simulink library "sm_motor_grader_lib"  (R2026a)
settings: Solver=VariableStepAuto
undefined symbols (not defined in the file): activeTestCmds, Art, Center, Circle, Driver, HMPST, LiftL, LiftR, LnL, LnR, Loads, Maneuver, motGradParams, Pin, RFL, RFR, RRL, RRR, SceneData, Side, Sphere, StrL, StrR, Tilt, X, Y, Z
libraries: sm_lib x219, nesl_utility x134, fl_lib x53, $bdroot x24, cvt_powertrain_lib x6, simulink_extras x5, grid_element x4, simulink x3, cvt_powertrain_lib_vnts x3, Driver_Long_Lat_Stanley x1, Maneuver_Get_Pose x1, SignalEditorBlockLib x1
(part 7 of 13)

== system sm_motor_grader_lib/Powertrain/Torque4 ==
  BusElementIn : Inport  PortName=Cmd  Element=vVeh
  BusElementIn1 : Inport  Port=2  PortName=m  Element=FrameR.Body.Ref.vx
  Gain : Gain  Gain=motGradParams.drivetrain.propGain
  Gain1 : Gain  Gain=motGradParams.drivetrain.integral
  Gain2 : Gain  Gain=4
  Integrator : Integrator
  Mechanical Rotational Reference : fl_lib/Mechanical/Rotational Elements/Mechanical Rotational Reference
  Simscape Bus : SimscapeBus  HierarchyStrings=RFL;RFR;RRL;RRR
  Simulink-PS Converter{,1..3} (4 alike) : nesl_utility/Simulink-PS Converter  PhysicalDomain=network_engine_domain  SubClassName=ps_input  LeftPortType=input  RightPortType=output  PseudoPeriodic=off  Frequencies=[]  NoiseDistribution=none  NoiseParameters=[]  Unit=1  AffineConversion=off  FilteringAndDerivatives=provide  SimscapeFilterOrder=1  InputFilterTimeConstant=0.001  UdotUserProvided=0
  Subtract : Sum  Inputs=+-
  Sum : Sum  Inputs=|++
  Torque Source FL : fl_lib/Mechanical/Mechanical Sources/Ideal Torque Source
  Torque Source FR : fl_lib/Mechanical/Mechanical Sources/Ideal Torque Source
  Torque Source RL : fl_lib/Mechanical/Mechanical Sources/Ideal Torque Source
  Torque Source RR : fl_lib/Mechanical/Mechanical Sources/Ideal Torque Source
  Dtr : PMIOPort  Side=Right
  Out Bus Element : Outport  PortName=meas  Element=trqDrv
  wires:
  BusElementIn/1 -> Subtract/1
  Subtract/1 -> Gain1/1, Gain/1
  Gain1/1 -> Integrator/1
  Gain/1 -> Sum/1
  Integrator/1 -> Sum/2
  Sum/1 -> Simulink-PS Converter1/1, Simulink-PS Converter/1, Gain2/1, Simulink-PS Converter2/1, Simulink-PS Converter3/1
  BusElementIn1/1 -> Subtract/2
  Gain2/1 -> Out Bus Element/1
  connections:
  Torque Source FL/RConn2 -- Torque Source FR/RConn2 -- Mechanical Rotational Reference/LConn1 -- Torque Source RR/RConn2 -- Torque Source RL/RConn2
  Simulink-PS Converter2/RConn1 -- Torque Source RL/RConn1
  Simulink-PS Converter/RConn1 -- Torque Source FL/RConn1
  Torque Source RL/LConn1 -- Simscape Bus/LConn3
  Simulink-PS Converter3/RConn1 -- Torque Source RR/RConn1
  Torque Source RR/LConn1 -- Simscape Bus/LConn4
  Simulink-PS Converter1/RConn1 -- Torque Source FR/RConn1
  Torque Source FL/LConn1 -- Simscape Bus/LConn1
  Torque Source FR/LConn1 -- Simscape Bus/LConn2
  Dtr/RConn1 -- Simscape Bus/RConn1

== system sm_motor_grader_lib/Surface/Bank ==
  Bank : grid_element/Grid  VariantControl=Grid  grid_x=SceneData.bank.grid.len  grid_y=SceneData.bank.grid.wid  grid_z=SceneData.bank.grid.dep  grid_line_width=SceneData.bank.grid.line_wid  grid_num_sq_x=SceneData.bank.grid.nsq_x  grid_num_sq_y=SceneData.bank.grid.nsq_y  grid_clr=SceneData.bank.grid.line_clr  plane_clr=SceneData.bank.grid.surf_clr  grid_opc=SceneData.bank.grid.line_opc  plane_opc=SceneData.bank.grid.surf_opc
  Grid : grid_element/Grid  VariantControl=Grid  grid_x=SceneData.grid.len  grid_y=SceneData.grid.wid  grid_z=SceneData.grid.dep  grid_line_width=SceneData.grid.line_wid  grid_num_sq_x=SceneData.grid.nsq_x  grid_num_sq_y=SceneData.grid.nsq_y  grid_clr=SceneData.grid.line_clr  plane_clr=SceneData.bank.grid.surf_clr  grid_opc=SceneData.grid.line_opc  plane_opc=SceneData.grid.surf_opc
  Grid Surface : sm_lib/Curves and Surfaces/Grid Surface  XGridVector=SceneData.bank.x_vec  XGridVectorUnits=m  YGridVector=SceneData.bank.y_vec  YGridVectorUnits=m  ZHeights=SceneData.bank.z_mat  ZHeightsUnits=m  GraphicType=None  GraphicVisPropType=SimpleVisualProperties  GraphicDiffuseColor=SceneData.bank.clr  GraphicOpacity=1  GraphicSpecularColor=[0.5 0.5 0.5 1.0]  GraphicAmbientColor=[0.15 0.15 0.15 1.0]  GraphicEmissiveColor=[0.0 0.0 0.0 1.0]  GraphicShininess=75
  Spline : sm_lib/Curves and Surfaces/Spline  DataPoints=[Maneuver.Trajectory.x.Value;Maneuver.Trajectory.y.Value;Maneuver.Trajectory.zbank.Value]'  DataPointsUnits=m  EndConditionType=Natural  GraphicType=FromGeometry  MarkerShape=Sphere  MarkerSize=10  GraphicVisPropType=SimpleVisualProperties  GraphicDiffuseColor=[0 0 0]  GraphicOpacity=1  GraphicSpecularColor=[0.5 0.5 0.5 1.0]  GraphicAmbientColor=[0.15 0.15 0.15 1.0]  GraphicEmissiveColor=[0.0 0.0 0.0 1.0]  GraphicShininess=75
  Transform Offset Bank : sm_lib/Frames and Transforms/Rigid Transform  RotationMethod=StandardAxis  FollAlignAxisA=+X  BaseAlignAxisA=+Y  FollAlignAxisB=+Y  BaseAlignAxisB=+Z  RotationStandardAxis=+X  RotationAngle=SceneData.bank.qBank  RotationAngleUnits=deg  RotationArbitraryAxis=[0 0 1]  RotationSequenceAxes=FollowerAxes  RotationSequence=XYX  RotationSequenceAngles=[0 0 0]  RotationSequenceAnglesUnits=deg  RotationMatrix=[1 0 0;0 1 0;0 0 1]  Quaternion=[1 0 0 0]  TranslationMethod=Cartesian  TranslationCartesianOffset=SceneData.bank.offset  TranslationCartesianOffsetUnits=m  TranslationStandardAxis=+X  TranslationStandardOffset=SceneData.grid.len/2-10  TranslationStandardOffsetUnits=m  TranslationROffset=0  TranslationROffsetUnits=m  TranslationThetaOffset=0  TranslationThetaOffsetUnits=deg  TranslationZOffset=0  TranslationZOffsetUnits=m
  Transform Offset Grid : sm_lib/Frames and Transforms/Rigid Transform  RotationMethod=None  FollAlignAxisA=+X  BaseAlignAxisA=+Y  FollAlignAxisB=+Y  BaseAlignAxisB=+Z  RotationStandardAxis=+Z  RotationAngle=0  RotationAngleUnits=deg  RotationArbitraryAxis=[0 0 1]  RotationSequenceAxes=FollowerAxes  RotationSequence=XYX  RotationSequenceAngles=[0 0 0]  RotationSequenceAnglesUnits=deg  RotationMatrix=[1 0 0;0 1 0;0 0 1]  Quaternion=[1 0 0 0]  TranslationMethod=StandardAxis  TranslationCartesianOffset=[0 0 0]  TranslationCartesianOffsetUnits=m  TranslationStandardAxis=+X  TranslationStandardOffset=SceneData.grid.len/2-10  TranslationStandardOffsetUnits=m  TranslationROffset=0  TranslationROffsetUnits=m  TranslationThetaOffset=0  TranslationThetaOffsetUnits=deg  TranslationZOffset=0  TranslationZOffsetUnits=m
  G : PMIOPort  Side=Right
  W : PMIOPort  Port=2  Side=Left
  connections:
  G/RConn1 -- Grid Surface/RConn1
  Transform Offset Grid/LConn1 -- Spline/LConn1 -- W/RConn1
  Grid/RConn1 -- Transform Offset Bank/LConn1 -- Grid Surface/LConn1 -- Transform Offset Grid/RConn1
  Bank/RConn1 -- Transform Offset Bank/RConn1

== system sm_motor_grader_lib/Surface/Grid ==
  Grid : grid_element/Grid  VariantControl=Grid  grid_x=SceneData.grid.len  grid_y=SceneData.grid.wid  grid_z=SceneData.grid.dep  grid_line_width=SceneData.grid.line_wid  grid_num_sq_x=SceneData.grid.nsq_x  grid_num_sq_y=SceneData.grid.nsq_y  grid_clr=SceneData.grid.line_clr  plane_clr=SceneData.grid.surf_clr  grid_opc=SceneData.grid.line_opc  plane_opc=SceneData.grid.surf_opc
  Infinite Plane : sm_lib/Curves and Surfaces/Infinite Plane  GraphicType=None  GraphicPlaneWidth=10  GraphicPlaneWidthUnits=m  GraphicPlaneHeight=10  GraphicPlaneHeightUnits=m  GraphicVisPropType=SimpleVisualProperties  GraphicDiffuseColor=[0.8 0.8 0.8]  GraphicOpacity=0.7  GraphicSpecularColor=[0.5 0.5 0.5 1.0]  GraphicAmbientColor=[0.15 0.15 0.15 1.0]  GraphicEmissiveColor=[0.0 0.0 0.0 1.0]  GraphicShininess=75
  Spline : sm_lib/Curves and Surfaces/Spline  DataPoints=[Maneuver.Trajectory.x.Value;Maneuver.Trajectory.y.Value;Maneuver.Trajectory.zgrid.Value]'  DataPointsUnits=m  EndConditionType=Natural  GraphicType=FromGeometry  MarkerShape=Sphere  MarkerSize=10  GraphicVisPropType=SimpleVisualProperties  GraphicDiffuseColor=[0 0 0]  GraphicOpacity=1  GraphicSpecularColor=[0.5 0.5 0.5 1.0]  GraphicAmbientColor=[0.15 0.15 0.15 1.0]  GraphicEmissiveColor=[0.0 0.0 0.0 1.0]  GraphicShininess=75
  Transform Offset Grid : sm_lib/Frames and Transforms/Rigid Transform  RotationMethod=None  FollAlignAxisA=+X  BaseAlignAxisA=+Y  FollAlignAxisB=+Y  BaseAlignAxisB=+Z  RotationStandardAxis=+Z  RotationAngle=0  RotationAngleUnits=deg  RotationArbitraryAxis=[0 0 1]  RotationSequenceAxes=FollowerAxes  RotationSequence=XYX  RotationSequenceAngles=[0 0 0]  RotationSequenceAnglesUnits=deg  RotationMatrix=[1 0 0;0 1 0;0 0 1]  Quaternion=[1 0 0 0]  TranslationMethod=StandardAxis  TranslationCartesianOffset=[0 0 0]  TranslationCartesianOffsetUnits=m  TranslationStandardAxis=+X  TranslationStandardOffset=SceneData.grid.len/2-10  TranslationStandardOffsetUnits=m  TranslationROffset=0  TranslationROffsetUnits=m  TranslationThetaOffset=0  TranslationThetaOffsetUnits=deg  TranslationZOffset=0  TranslationZOffsetUnits=m
  G : PMIOPort  Side=Right
  W : PMIOPort  Port=2  Side=Left
  connections:
  Grid/RConn1 -- Transform Offset Grid/RConn1
  W/RConn1 -- Spline/LConn1 -- Transform Offset Grid/LConn1 -- Infinite Plane/LConn1
  G/RConn1 -- Infinite Plane/RConn1

== system sm_motor_grader_lib/Surface/Parked ==
  Grid : grid_element/Grid  VariantControl=Grid  grid_x=SceneData.park.len  grid_y=SceneData.park.wid  grid_z=SceneData.park.dep  grid_line_width=SceneData.park.line_wid  grid_num_sq_x=SceneData.park.nsq_x  grid_num_sq_y=SceneData.park.nsq_y  grid_clr=SceneData.park.line_clr  plane_clr=SceneData.park.surf_clr  grid_opc=SceneData.park.line_opc  plane_opc=SceneData.park.surf_opc
  Infinite Plane : sm_lib/Curves and Surfaces/Infinite Plane  GraphicType=None  GraphicPlaneWidth=10  GraphicPlaneWidthUnits=m  GraphicPlaneHeight=10  GraphicPlaneHeightUnits=m  GraphicVisPropType=SimpleVisualProperties  GraphicDiffuseColor=[0.8 0.8 0.8]  GraphicOpacity=0.7  GraphicSpecularColor=[0.5 0.5 0.5 1.0]  GraphicAmbientColor=[0.15 0.15 0.15 1.0]  GraphicEmissiveColor=[0.0 0.0 0.0 1.0]  GraphicShininess=75
  Transform Offset Grid : sm_lib/Frames and Transforms/Rigid Transform  RotationMethod=None  FollAlignAxisA=+X  BaseAlignAxisA=+Y  FollAlignAxisB=+Y  BaseAlignAxisB=+Z  RotationStandardAxis=+Z  RotationAngle=0  RotationAngleUnits=deg  RotationArbitraryAxis=[0 0 1]  RotationSequenceAxes=FollowerAxes  RotationSequence=XYX  RotationSequenceAngles=[0 0 0]  RotationSequenceAnglesUnits=deg  RotationMatrix=[1 0 0;0 1 0;0 0 1]  Quaternion=[1 0 0 0]  TranslationMethod=StandardAxis  TranslationCartesianOffset=[0 0 0]  TranslationCartesianOffsetUnits=m  TranslationStandardAxis=+X  TranslationStandardOffset=SceneData.park.len/2-10  TranslationStandardOffsetUnits=m  TranslationROffset=0  TranslationROffsetUnits=m  TranslationThetaOffset=0  TranslationThetaOffsetUnits=deg  TranslationZOffset=0  TranslationZOffsetUnits=m
  G : PMIOPort  Side=Right
  W : PMIOPort  Port=2  Side=Left
  connections:
  G/RConn1 -- Infinite Plane/RConn1
  Infinite Plane/LConn1 -- Transform Offset Grid/LConn1 -- W/RConn1
  Grid/RConn1 -- Transform Offset Grid/RConn1

== system sm_motor_grader_lib/Surface/Terrain ==
  Grid Surface : sm_lib/Curves and Surfaces/Grid Surface  XGridVector=SceneData.terrain.x  XGridVectorUnits=m  YGridVector=SceneData.terrain.y  YGridVectorUnits=m  ZHeights=SceneData.terrain.h  ZHeightsUnits=m  GraphicType=FromGeometry  GraphicVisPropType=SimpleVisualProperties  GraphicDiffuseColor=SceneData.terrain.clr  GraphicOpacity=1  GraphicSpecularColor=[0.5 0.5 0.5 1.0]  GraphicAmbientColor=[0.15 0.15 0.15 1.0]  GraphicEmissiveColor=[0.0 0.0 0.0 1.0]  GraphicShininess=75
  Spline : sm_lib/Curves and Surfaces/Spline  DataPoints=[Maneuver.Trajectory.x.Value;Maneuver.Trajectory.y.Value;Maneuver.Trajectory.zterrain.Value]'  DataPointsUnits=m  EndConditionType=Natural  GraphicType=FromGeometry  MarkerShape=Sphere  MarkerSize=10  GraphicVisPropType=SimpleVisualProperties  GraphicDiffuseColor=[0 0 0]  GraphicOpacity=1  GraphicSpecularColor=[0.5 0.5 0.5 1.0]  GraphicAmbientColor=[0.15 0.15 0.15 1.0]  GraphicEmissiveColor=[0.0 0.0 0.0 1.0]  GraphicShininess=75
  G : PMIOPort  Side=Right
  W : PMIOPort  Port=2  Side=Left
  connections:
  Grid Surface/RConn1 -- G/RConn1
  W/RConn1 -- Spline/LConn1 -- Grid Surface/LConn1

== system sm_motor_grader_lib/Actuation/Actuator LiftL/Position ==
  pCmd : Inport
  pMeas : Inport  Port=2
  mLiftL : Inport  Port=3
  Terminator : Terminator
  Terminator1 : Terminator
  Terminator3 : Terminator
  R : PMIOPort  Side=Right
  wires:
  pCmd/1 -> Terminator1/1
  pMeas/1 -> Terminator/1
  mLiftL/1 -> Terminator3/1

== system sm_motor_grader_lib/Actuation/Actuator LiftL/Shaft ==
  note: Cylinder Floats
  pCmd : Inport
  pMeas : Inport  Port=2
  mLiftL : Inport  Port=3
  Compare To Constant2 : simulink/Logic and Bit Operations/Compare To Constant  relop===  const=1  OutDataTypeStr=boolean
  Constant : Constant  Value=0
  Force Source LiftL : fl_lib/Mechanical/Mechanical Sources/Ideal Force Source
  Gain : Gain  Gain=motGradParams.bladeLift.propGain
  Gain1 : Gain  Gain=motGradParams.bladeLift.integral
  Gain2 : Gain  Gain=motGradParams.bladeLift.derivative
  Integrator : Integrator  ExternalReset=either
  Mechanical Translational Reference : fl_lib/Mechanical/Translational Elements/Mechanical Translational Reference
  Simulink-PS Converter : nesl_utility/Simulink-PS Converter  PhysicalDomain=network_engine_domain  SubClassName=ps_input  LeftPortType=input  RightPortType=output  PseudoPeriodic=off  Frequencies=[]  NoiseDistribution=none  NoiseParameters=[]  Unit=1  AffineConversion=off  FilteringAndDerivatives=provide  SimscapeFilterOrder=1  InputFilterTimeConstant=0.001  UdotUserProvided=0
  Subtract : Sum  Inputs=+-
  Sum1 : Sum  Inputs=+++
  Switch : Switch  Criteria=u2 > Threshold  ZeroCross=off  SaturateOnIntegerOverflow=off  InputSameDT=off
  Transfer Fcn : TransferFcn  Numerator=[1 0]  Denominator=[0.01 1]
  Transfer Fcn (with initial outputs) : simulink_extras/Additional Linear/Transfer Fcn (with initial outputs)  N=[1]  D="[0.01  1]"  Y0=motGradParams.bladeLift.leftInitPos  U0=motGradParams.bladeLift.leftInitPos
  R : PMIOPort  Side=Right
  wires:
  Gain2/1 -> Transfer Fcn/1
  Integrator/1 -> Sum1/2
  Transfer Fcn/1 -> Sum1/3
  Gain/1 -> Sum1/1
  Subtract/1 -> Gain/1, Gain1/1, Gain2/1
  Gain1/1 -> Integrator/1
  Transfer Fcn (with initial outputs)/1 -> Subtract/2
  Sum1/1 -> Switch/3  "Force Command"
  Constant/1 -> Switch/1
  pMeas/1 -> Transfer Fcn (with initial outputs)/1
  pCmd/1 -> Subtract/1
  Switch/1 -> Simulink-PS Converter/1
  mLiftL/1 -> Switch/2, Compare To Constant2/1
  Compare To Constant2/1 -> Integrator/2
  connections:
  Force Source LiftL/RConn2 -- Mechanical Translational Reference/LConn1
  R/RConn1 -- Force Source LiftL/LConn1
  Simulink-PS Converter/RConn1 -- Force Source LiftL/RConn1

== system sm_motor_grader_lib/Actuation/Actuator LiftR/Position ==
  pCmd : Inport
  pMeas : Inport  Port=2
  mLiftR : Inport  Port=3
  Terminator : Terminator
  Terminator1 : Terminator
  Terminator3 : Terminator
  R : PMIOPort  Side=Right
  wires:
  pCmd/1 -> Terminator1/1
  pMeas/1 -> Terminator/1
  mLiftR/1 -> Terminator3/1

== system sm_motor_grader_lib/Actuation/Actuator LiftR/Shaft ==
  note: Cylinder Floats
  pCmd : Inport
  pMeas : Inport  Port=2
  mLiftR : Inport  Port=3
  Compare To Constant2 : simulink/Logic and Bit Operations/Compare To Constant  relop===  const=1  OutDataTypeStr=boolean
  Constant : Constant  Value=0
  Force Source : fl_lib/Mechanical/Mechanical Sources/Ideal Force Source
  Gain : Gain  Gain=motGradParams.bladeLift.propGain
  Gain1 : Gain  Gain=motGradParams.bladeLift.integral
  Gain2 : Gain  Gain=motGradParams.bladeLift.derivative
  Integrator : Integrator  ExternalReset=either
  Mechanical Translational Reference1 : fl_lib/Mechanical/Translational Elements/Mechanical Translational Reference
  Simulink-PS Converter1 : nesl_utility/Simulink-PS Converter  PhysicalDomain=network_engine_domain  SubClassName=ps_input  LeftPortType=input  RightPortType=output  PseudoPeriodic=off  Frequencies=[]  NoiseDistribution=none  NoiseParameters=[]  Unit=1  AffineConversion=off  FilteringAndDerivatives=provide  SimscapeFilterOrder=1  InputFilterTimeConstant=0.001  UdotUserProvided=0
  Subtract : Sum  Inputs=+-
  Sum1 : Sum  Inputs=+++
  Switch : Switch  Criteria=u2 > Threshold  ZeroCross=off  SaturateOnIntegerOverflow=off  InputSameDT=off
  Transfer Fcn : TransferFcn  Numerator=[1 0]  Denominator=[0.01 1]
  Transfer Fcn (with initial outputs) : simulink_extras/Additional Linear/Transfer Fcn (with initial outputs)  N=[1]  D="[0.01  1]"  Y0=motGradParams.bladeLift.rightInitPos  U0=motGradParams.bladeLift.rightInitPos
  R : PMIOPort  Side=Right
  wires:
  Gain1/1 -> Integrator/1
  Gain/1 -> Sum1/1
  Transfer Fcn/1 -> Sum1/3
  Integrator/1 -> Sum1/2
  Gain2/1 -> Transfer Fcn/1
  Subtract/1 -> Gain/1, Gain2/1, Gain1/1
  Constant/1 -> Switch/1
  pMeas/1 -> Transfer Fcn (with initial outputs)/1
  Sum1/1 -> Switch/3  "Force Command"
  Transfer Fcn (with initial outputs)/1 -> Subtract/2
  pCmd/1 -> Subtract/1
  Switch/1 -> Simulink-PS Converter1/1
  mLiftR/1 -> Switch/2, Compare To Constant2/1
  Compare To Constant2/1 -> Integrator/2
  connections:
  Force Source/LConn1 -- R/RConn1
  Simulink-PS Converter1/RConn1 -- Force Source/RConn1
  Force Source/RConn2 -- Mechanical Translational Reference1/LConn1

== system sm_motor_grader_lib/Actuation/Actuator Pinion/Position ==
  qCmd : Inport
  qMeas : Inport  Port=2
  Terminator : Terminator
  Terminator1 : Terminator
  R : PMIOPort  Side=Right
  wires:
  qCmd/1 -> Terminator/1
  qMeas/1 -> Terminator1/1

== system sm_motor_grader_lib/Actuation/Actuator Pinion/Shaft ==
  qCmd : Inport
  qMeas : Inport  Port=2
  Gain : Gain  Gain=motGradParams.circleRot.propGain
  Gain1 : Gain  Gain=motGradParams.circleRot.integral
  Gain2 : Gain  Gain=motGradParams.circleRot.derivative
  Integrator : Integrator  InitialCondition=motGradParams.circleRot.initPos
  Mechanical Rotational Reference : fl_lib/Mechanical/Rotational Elements/Mechanical Rotational Reference
  Simulink-PS Converter2 : nesl_utility/Simulink-PS Converter  PhysicalDomain=network_engine_domain  SubClassName=ps_input  LeftPortType=input  RightPortType=output  PseudoPeriodic=off  Frequencies=[]  NoiseDistribution=none  NoiseParameters=[]  Unit=1  AffineConversion=off  FilteringAndDerivatives=provide  SimscapeFilterOrder=1  InputFilterTimeConstant=0.001  UdotUserProvided=0
  Subtract : Sum  Inputs=+-
  Sum : Sum  Inputs=+++
  Torque Source : fl_lib/Mechanical/Mechanical Sources/Ideal Torque Source
  Transfer Fcn : TransferFcn  Numerator=[1 0]  Denominator=[0.01 1]
  Transfer Fcn (with initial outputs) : simulink_extras/Additional Linear/Transfer Fcn (with initial outputs)  N=[1]  D="[0.01  1]"  Y0=motGradParams.circleRot.initPos  U0=motGradParams.circleRot.initPos
  R : PMIOPort  Side=Right
  wires:
  Integrator/1 -> Sum/2
  Transfer Fcn/1 -> Sum/3
  Gain2/1 -> Transfer Fcn/1
  Gain1/1 -> Integrator/1
  Gain/1 -> Sum/1
  Transfer Fcn (with initial outputs)/1 -> Subtract/2
  Subtract/1 -> Gain1/1, Gain2/1, Gain/1
  qMeas/1 -> Transfer Fcn (with initial outputs)/1
  qCmd/1 -> Subtract/1
  Sum/1 -> Simulink-PS Converter2/1
  connections:
  Simulink-PS Converter2/RConn1 -- Torque Source/RConn1
  Torque Source/LConn1 -- R/RConn1
  Torque Source/RConn2 -- Mechanical Rotational Reference/LConn1

== system sm_motor_grader_lib/Blade/Blade/Ground Forces ==
  Loads : Subsystem  VariantControl=Loads
      settings: PortSchema="{\"entries\":[{\"content\":{\"sides\":[{\"content\":{\"connectorIds\":[\"LConn1\",\"LConn2\"]},\"type\":\"ConnectorPlacement.EquallySpacedRectSide\",\"uuid\":\"8c9ce02f-c33d-45a2-bc09-c637b621747d\"},{\"content\":{\"connectorIds\":[\"Out1\",\"RConn1\"],\"side\":\"RIGHT\"},\"type\":\"ConnectorPlacement.EquallySpacedRectSide\",\"uuid\":\"ca505da9-45b8-4d49-8a5b-fa2b61b33c10\"},{\"content\":{\"side\":\"TOP\"},\"type\":\"ConnectorPlacement.EquallySpacedRectSide\",\"uuid\":\"0ba4068c-c021-4d14-9fe5-8ec7e3b7739f\"},{\"content\":{\"connectorIds\":[\"RConn2\"],\"side\":\"BOTTOM\"},\"type\":\"ConnectorPlacement.EquallySpacedRectSide\",\"uuid\":\"fb7e3d81-efbb-4c28-8e06-39679b9f1ef2\"}]},\"type\":\"ConnectorPlacement.EquallySpacedConnector\",\"uuid\":\"f3b68a2d-a585-40c4-a7f5-e74692c73c61\"}],\"packageUris\":[\"http://schema.mathworks.com/mf0/Connector/R2020b\"],\"version\":\"1.0\"}"
  None : Subsystem  VariantControl=None
      settings: PortSchema="{\"entries\":[{\"content\":{\"sides\":[{\"content\":{\"connectorIds\":[\"LConn1\",\"LConn2\"]},\"type\":\"ConnectorPlacement.EquallySpacedRectSide\",\"uuid\":\"8c9ce02f-c33d-45a2-bc09-c637b621747d\"},{\"content\":{\"connectorIds\":[\"Out1\",\"RConn1\"],\"side\":\"RIGHT\"},\"type\":\"ConnectorPlacement.EquallySpacedRectSide\",\"uuid\":\"ca505da9-45b8-4d49-8a5b-fa2b61b33c10\"},{\"content\":{\"side\":\"TOP\"},\"type\":\"ConnectorPlacement.EquallySpacedRectSide\",\"uuid\":\"0ba4068c-c021-4d14-9fe5-8ec7e3b7739f\"},{\"content\":{\"connectorIds\":[\"RConn2\"],\"side\":\"BOTTOM\"},\"type\":\"ConnectorPlacement.EquallySpacedRectSide\",\"uuid\":\"fb7e3d81-efbb-4c28-8e06-39679b9f1ef2\"}]},\"type\":\"ConnectorPlacement.EquallySpacedConnector\",\"uuid\":\"f3b68a2d-a585-40c4-a7f5-e74692c73c61\"}],\"packageUris\":[\"http://schema.mathworks.com/mf0/Connector/R2020b\"],\"version\":\"1.0\"}"
  Normal : Subsystem  VariantControl=Normal
      settings: PortSchema="{\"entries\":[{\"content\":{\"sides\":[{\"content\":{\"connectorIds\":[\"LConn1\",\"LConn2\"]},\"type\":\"ConnectorPlacement.EquallySpacedRectSide\",\"uuid\":\"8c9ce02f-c33d-45a2-bc09-c637b621747d\"},{\"content\":{\"connectorIds\":[\"Out1\",\"RConn1\"],\"side\":\"RIGHT\"},\"type\":\"ConnectorPlacement.EquallySpacedRectSide\",\"uuid\":\"ca505da9-45b8-4d49-8a5b-fa2b61b33c10\"},{\"content\":{\"side\":\"TOP\"},\"type\":\"ConnectorPlacement.EquallySpacedRectSide\",\"uuid\":\"0ba4068c-c021-4d14-9fe5-8ec7e3b7739f\"},{\"content\":{\"connectorIds\":[\"RConn2\"],\"side\":\"BOTTOM\"},\"type\":\"ConnectorPlacement.EquallySpacedRectSide\",\"uuid\":\"fb7e3d81-efbb-4c28-8e06-39679b9f1ef2\"}]},\"type\":\"ConnectorPlacement.EquallySpacedConnector\",\"uuid\":\"f3b68a2d-a585-40c4-a7f5-e74692c73c61\"}],\"packageUris\":[\"http://schema.mathworks.com/mf0/Connector/R2020b\"],\"version\":\"1.0\"}"
  Ctr : PMIOPort  Side=Left
  R : PMIOPort  Port=2  Side=Left
  L : PMIOPort  Port=3  Side=Right
  G : PMIOPort  Port=4  Side=Right
  m : Outport

== system sm_motor_grader_lib/Blade/Shift Actuator/Actuator ==
  p : Inport
  Position : Subsystem  VariantControl=Position
      mask Display: image('sm_motor_grader_cyljoint_Position_IMAGE.png')
  Shaft : Subsystem  VariantControl=Shaft
      mask Display: image('sm_motor_grader_cyljoint_Shaft_IMAGE.png')
  R : PMIOPort  Side=Left
  B : PMIOPort  Port=2  Side=Left
  F : PMIOPort  Port=3  Side=Right
  m : Outport

== system sm_motor_grader_lib/Blade/Shift Actuator/Cyilnder ==
  Blade Shift Cyl : sm_lib/Body Elements/File Solid  ExtGeomFileName=BladeSideShiftCylinder.step  UnitType=FromFile  ExtGeomFileUnits=m  StepReaderType=HEX  ExportConvexHullGeometry=off  InertiaType=CalculateFromGeometry  BasedOnType=Mass  Density=1000  DensityUnits=kg/m^3  Mass=motGradParams.bladeSideShift.cyl.mass  MassUnits=kg  CenterOfMass=[0 0 0]  CenterOfMassUnits=m  MomentsOfInertia=[1 1 1]  MomentsOfInertiaUnits=kg*m^2  ProductsOfInertia=[0 0 0]  ProductsOfInertiaUnits=kg*m^2  GraphicType=FromGeometry  MarkerShape=Sphere  MarkerSize=10  GraphicVisPropType=SimpleVisualProperties  GraphicDiffuseColor=mtrgrd.clr.blade_shift_cyl  GraphicOpacity=1  GraphicSpecularColor=[0.5 0.5 0.5 1.0]  GraphicAmbientColor=[0.15 0.15 0.15 1.0]  GraphicEmissiveColor=[0.0 0.0 0.0 1.0]  GraphicShininess=75  DoExposeReferenceFrame=off  SerializedFrames=<Frames><Frame><Id>Frame1</Id><Value><Name>BladeTiltFrame</Name><Origin><Source>GeometricFeature</Source><FeatureName>circular curve 13</FeatureName></Origin><PrimaryAxis><DefinedDirection>+Z</DefinedDirection><Source>ReferenceFrame</Source><SourceDirection>+Z</SourceDirection><FeatureName></FeatureName></PrimaryAxis><SecondaryAxis><DefinedDirection>+X</DefinedDirection><Source>ReferenceFrame</Source><SourceDirection>+X</SourceDirection><FeatureName></FeatureName></SecondaryAxis></Value></Frame><Frame><Id>Frame2</Id><Value><Name>BladeTiltRod</Name><Origin><Source>GeometricFeature</Source><FeatureName>planar surface 12</FeatureName></Origin><PrimaryAxis><DefinedDirection>-Z</DefinedDirection><Source>GeometricFeature</Source><SourceDirection>+Z</SourceDirection><FeatureName>segment 23</FeatureName></PrimaryAxis><SecondaryAxis><DefinedDirection>+X</DefinedDirection><Source>ReferenceFrame</Source><SourceDirection>+X</SourceDirection><FeatureName></FeatureName></SecondaryAxis></Value></Frame></Frames>
  Transform Cyl Joint : sm_lib/Frames and Transforms/Rigid Transform  RotationMethod=StandardAxis  FollAlignAxisA=+X  BaseAlignAxisA=+Y  FollAlignAxisB=+Y  BaseAlignAxisB=+Z  RotationStandardAxis=+Y  RotationAngle=90  RotationAngleUnits=deg  RotationArbitraryAxis=[0 0 1]  RotationSequenceAxes=FollowerAxes  RotationSequence=XYX  RotationSequenceAngles=[0 0 0]  RotationSequenceAnglesUnits=deg  RotationMatrix=[1 0 0;0 1 0;0 0 1]  Quaternion=[1 0 0 0]  TranslationMethod=None  TranslationCartesianOffset=[0 0 0]  TranslationCartesianOffsetUnits=m  TranslationStandardAxis=+Z  TranslationStandardOffset=0  TranslationStandardOffsetUnits=m  TranslationROffset=0  TranslationROffsetUnits=m  TranslationThetaOffset=0  TranslationThetaOffsetUnits=deg  TranslationZOffset=0  TranslationZOffsetUnits=m
  B : PMIOPort  Side=Left
  F : PMIOPort  Port=2  Side=Right
  connections:
  Transform Cyl Joint/LConn1 -- Blade Shift Cyl/LConn1
  F/RConn1 -- Blade Shift Cyl/RConn1
  Transform Cyl Joint/RConn1 -- B/RConn1

== system sm_motor_grader_lib/Blade/Shift Actuator/Rod ==
  Blade Shift Rod : sm_lib/Body Elements/File Solid  ExtGeomFileName=BladeSideShiftRod.step  UnitType=FromFile  ExtGeomFileUnits=m  StepReaderType=HEX  ExportConvexHullGeometry=off  InertiaType=CalculateFromGeometry  BasedOnType=Mass  Density=1000  DensityUnits=kg/m^3  Mass=motGradParams.bladeSideShift.rod.mass  MassUnits=kg  CenterOfMass=[0 0 0]  CenterOfMassUnits=m  MomentsOfInertia=[1 1 1]  MomentsOfInertiaUnits=kg*m^2  ProductsOfInertia=[0 0 0]  ProductsOfInertiaUnits=kg*m^2  GraphicType=FromGeometry  MarkerShape=Sphere  MarkerSize=10  GraphicVisPropType=SimpleVisualProperties  GraphicDiffuseColor=mtrgrd.clr.blade_shift_rod  GraphicOpacity=1  GraphicSpecularColor=[0.5 0.5 0.5 1.0]  GraphicAmbientColor=[0.15 0.15 0.15 1.0]  GraphicEmissiveColor=[0.0 0.0 0.0 1.0]  GraphicShininess=75  DoExposeReferenceFrame=off  SerializedFrames=<Frames><Frame><Id>Frame1</Id><Value><Name>BladeSideShiftCyl</Name><Origin><Source>GeometricFeature</Source><FeatureName>planar surface 7</FeatureName></Origin><PrimaryAxis><DefinedDirection>-Z</DefinedDirection><Source>GeometricFeature</Source><SourceDirection>+Z</SourceDirection><FeatureName>segment 21</FeatureName></PrimaryAxis><SecondaryAxis><DefinedDirection>+X</DefinedDirection><Source>ReferenceFrame</Source><SourceDirection>+Z</SourceDirection><FeatureName></FeatureName></SecondaryAxis></Value></Frame><Frame><Id>Frame2</Id><Value><Name>Blade</Name><Origin><Source>GeometricFeature</Source><FeatureName>circular curve 9</FeatureName></Origin><PrimaryAxis><DefinedDirection>+Z</DefinedDirection><Source>GeometricFeature</Source><SourceDirection>+Z</SourceDirection><FeatureName>segment 19</FeatureName></PrimaryAxis><SecondaryAxis><DefinedDirection>+X</DefinedDirection><Source>ReferenceFrame</Source><SourceDirection>+Z</SourceDirection><FeatureName></FeatureName></SecondaryAxis></Value></Frame></Frames>
  Transform Rod Joint : sm_lib/Frames and Transforms/Rigid Transform  RotationMethod=StandardAxis  FollAlignAxisA=+X  BaseAlignAxisA=+Y  FollAlignAxisB=+Y  BaseAlignAxisB=+Z  RotationStandardAxis=+X  RotationAngle=90  RotationAngleUnits=deg  RotationArbitraryAxis=[0 0 1]  RotationSequenceAxes=FollowerAxes  RotationSequence=XYX  RotationSequenceAngles=[0 0 0]  RotationSequenceAnglesUnits=deg  RotationMatrix=[1 0 0;0 1 0;0 0 1]  Quaternion=[1 0 0 0]  TranslationMethod=None  TranslationCartesianOffset=[0 0 0]  TranslationCartesianOffsetUnits=m  TranslationStandardAxis=+Z  TranslationStandardOffset=0  TranslationStandardOffsetUnits=m  TranslationROffset=0  TranslationROffsetUnits=m  TranslationThetaOffset=0  TranslationThetaOffsetUnits=deg  TranslationZOffset=0  TranslationZOffsetUnits=m
  B : PMIOPort  Side=Left
  F : PMIOPort  Port=2  Side=Right
  connections:
  Transform Rod Joint/LConn1 -- Blade Shift Rod/RConn1
  Transform Rod Joint/RConn1 -- F/RConn1
  B/RConn1 -- Blade Shift Rod/LConn1

== system sm_motor_grader_lib/Blade/Tilt Actuator/Actuator ==
  p : Inport
  Position : Subsystem  VariantControl=Position
      mask Display: image('sm_motor_grader_cyljoint_Position_IMAGE.png')
  Shaft : Subsystem  VariantControl=Shaft
      mask Display: image('sm_motor_grader_cyljoint_Shaft_IMAGE.png')
  R : PMIOPort  Side=Left
  B : PMIOPort  Port=2  Side=Left
  F : PMIOPort  Port=3  Side=Right
  m : Outport

== system sm_motor_grader_lib/Blade/Tilt Actuator/Cylinder ==
  Blade Tilt Cyilnder : sm_lib/Body Elements/File Solid  ExtGeomFileName=BladeTiltCyl.step  UnitType=FromFile  ExtGeomFileUnits=m  StepReaderType=HEX  ExportConvexHullGeometry=off  InertiaType=CalculateFromGeometry  BasedOnType=Mass  Density=1000  DensityUnits=kg/m^3  Mass=motGradParams.bladeTilt.cyl.mass  MassUnits=kg  CenterOfMass=[0 0 0]  CenterOfMassUnits=m  MomentsOfInertia=[1 1 1]  MomentsOfInertiaUnits=kg*m^2  ProductsOfInertia=[0 0 0]  ProductsOfInertiaUnits=kg*m^2  GraphicType=FromGeometry  MarkerShape=Sphere  MarkerSize=10  GraphicVisPropType=SimpleVisualProperties  GraphicDiffuseColor=mtrgrd.clr.blade_tilt_cyl  GraphicOpacity=1  GraphicSpecularColor=[0.5 0.5 0.5 1.0]  GraphicAmbientColor=[0.15 0.15 0.15 1.0]  GraphicEmissiveColor=[0.0 0.0 0.0 1.0]  GraphicShininess=75  DoExposeReferenceFrame=off  SerializedFrames=<Frames><Frame><Id>Frame1</Id><Value><Name>CircleFrame</Name><Origin><Source>GeometricFeature</Source><FeatureName>circular curve 53</FeatureName></Origin><PrimaryAxis><DefinedDirection>+Z</DefinedDirection><Source>GeometricFeature</Source><SourceDirection>+Z</SourceDirection><FeatureName>segment 32</FeatureName></PrimaryAxis><SecondaryAxis><DefinedDirection>-Y</DefinedDirection><Source>GeometricFeature</Source><SourceDirection>+X</SourceDirection><FeatureName>segment 29</FeatureName></SecondaryAxis></Value></Frame><Frame><Id>Frame2</Id><Value><Name>BladeTiltRod</Name><Origin><Source>GeometricFeature</Source><FeatureName>planar surface 9</FeatureName></Origin><PrimaryAxis><DefinedDirection>+Z</DefinedDirection><Source>GeometricFeature</Source><SourceDirection>+Z</SourceDirection><FeatureName>segment 5</FeatureName></PrimaryAxis><SecondaryAxis><DefinedDirection>+X</DefinedDirection><Source>GeometricFeature</Source><SourceDirection>+X</SourceDirection><FeatureName>segment 11</FeatureName></SecondaryAxis></Value></Frame></Frames>
  Rigid Transform1 : sm_lib/Frames and Transforms/Rigid Transform  RotationMethod=StandardAxis  FollAlignAxisA=+X  BaseAlignAxisA=+Y  FollAlignAxisB=+Y  BaseAlignAxisB=+Z  RotationStandardAxis=+X  RotationAngle=90  RotationAngleUnits=deg  RotationArbitraryAxis=[0 0 1]  RotationSequenceAxes=FollowerAxes  RotationSequence=XYX  RotationSequenceAngles=[0 0 0]  RotationSequenceAnglesUnits=deg  RotationMatrix=[1 0 0;0 1 0;0 0 1]  Quaternion=[1 0 0 0]  TranslationMethod=None  TranslationCartesianOffset=[0 0 0]  TranslationCartesianOffsetUnits=m  TranslationStandardAxis=+Z  TranslationStandardOffset=0  TranslationStandardOffsetUnits=m  TranslationROffset=0  TranslationROffsetUnits=m  TranslationThetaOffset=0  TranslationThetaOffsetUnits=deg  TranslationZOffset=0  TranslationZOffsetUnits=m
  B : PMIOPort  Side=Left
  F : PMIOPort  Port=2  Side=Right
  connections:
  Rigid Transform1/LConn1 -- Blade Tilt Cyilnder/LConn1
  F/RConn1 -- Blade Tilt Cyilnder/RConn1
  B/RConn1 -- Rigid Transform1/RConn1

== system sm_motor_grader_lib/Blade/Tilt Actuator/Rod ==
  Blade Tilt Rod : sm_lib/Body Elements/File Solid  ExtGeomFileName=BladeTiltRod.step  UnitType=FromFile  ExtGeomFileUnits=m  StepReaderType=HEX  ExportConvexHullGeometry=off  InertiaType=CalculateFromGeometry  BasedOnType=Mass  Density=1000  DensityUnits=kg/m^3  Mass=motGradParams.bladeTilt.rod.mass  MassUnits=kg  CenterOfMass=[0 0 0]  CenterOfMassUnits=m  MomentsOfInertia=[1 1 1]  MomentsOfInertiaUnits=kg*m^2  ProductsOfInertia=[0 0 0]  ProductsOfInertiaUnits=kg*m^2  GraphicType=FromGeometry  MarkerShape=Sphere  MarkerSize=10  GraphicVisPropType=SimpleVisualProperties  GraphicDiffuseColor=mtrgrd.clr.blade_tilt_rod  GraphicOpacity=1  GraphicSpecularColor=[0.5 0.5 0.5 1.0]  GraphicAmbientColor=[0.15 0.15 0.15 1.0]  GraphicEmissiveColor=[0.0 0.0 0.0 1.0]  GraphicShininess=75  DoExposeReferenceFrame=off  SerializedFrames=<Frames><Frame><Id>Frame1</Id><Value><Name>BladeTiltCyl</Name><Origin><Source>GeometricFeature</Source><FeatureName>circular curve 1</FeatureName></Origin><PrimaryAxis><DefinedDirection>+Z</DefinedDirection><Source>GeometricFeature</Source><SourceDirection>+Z</SourceDirection><FeatureName>segment 1</FeatureName></PrimaryAxis><SecondaryAxis><DefinedDirection>-Y</DefinedDirection><Source>GeometricFeature</Source><SourceDirection>+X</SourceDirection><FeatureName>segment 4</FeatureName></SecondaryAxis></Value></Frame><Frame><Id>Frame2</Id><Value><Name>BladeTiltFrame</Name><Origin><Source>GeometricFeature</Source><FeatureName>circular curve 10</FeatureName></Origin><PrimaryAxis><DefinedDirection>-Z</DefinedDirection><Source>GeometricFeature</Source><SourceDirection>+Z</SourceDirection><FeatureName>segment 4</FeatureName></PrimaryAxis><SecondaryAxis><DefinedDirection>-Y</DefinedDirection><Source>GeometricFeature</Source><SourceDirection>+X</SourceDirection><FeatureName>segment 1</FeatureName></SecondaryAxis></Value></Frame></Frames>
  Transform Rod Joint : sm_lib/Frames and Transforms/Rigid Transform  RotationMethod=StandardAxis  FollAlignAxisA=+X  BaseAlignAxisA=+Y  FollAlignAxisB=+Y  BaseAlignAxisB=+Z  RotationStandardAxis=+X  RotationAngle=90  RotationAngleUnits=deg  RotationArbitraryAxis=[0 0 1]  RotationSequenceAxes=FollowerAxes  RotationSequence=XYX  RotationSequenceAngles=[0 0 0]  RotationSequenceAnglesUnits=deg  RotationMatrix=[1 0 0;0 1 0;0 0 1]  Quaternion=[1 0 0 0]  TranslationMethod=None  TranslationCartesianOffset=[0 0 0]  TranslationCartesianOffsetUnits=m  TranslationStandardAxis=+Z  TranslationStandardOffset=0  TranslationStandardOffsetUnits=m  TranslationROffset=0  TranslationROffsetUnits=m  TranslationThetaOffset=0  TranslationThetaOffsetUnits=deg  TranslationZOffset=0  TranslationZOffsetUnits=m
  B : PMIOPort  Side=Left
  F : PMIOPort  Port=2  Side=Right
  connections:
  B/RConn1 -- Blade Tilt Rod/LConn1
  Blade Tilt Rod/RConn1 -- Transform Rod Joint/LConn1
  F/RConn1 -- Transform Rod Joint/RConn1

== system sm_motor_grader_lib/Control/Closed Loop/None ==
  Bus Creator{,2..4} (4 alike) : BusCreator  Inputs=2
  Bus Creator1 : BusCreator  Inputs=4
  Constant{1..2,4,6} (4 alike) : Constant  Value=0
  Constant3 : Constant
  Constant5 : Constant
  Constant7 : Constant
  Ramp : simulink/Sources/Ramp  slope=0.5  start=0.5  InitialOutput=0
  Saturation : Saturate  UpperLimit=1  LowerLimit=0  ZeroCross=off
  Ovr : Outport  VectorParamsAs1DForOutWhenUnconnected=off
  wires:
  Bus Creator1/1 -> Ovr/1
  Constant1/1 -> Bus Creator/1  "offset"
  Saturation/1 -> Bus Creator/2  "gain"
  Constant6/1 -> Bus Creator4/1  "offset"
  Constant7/1 -> Bus Creator4/2  "gain"
  Constant5/1 -> Bus Creator3/2  "gain"
  Constant4/1 -> Bus Creator3/1  "offset"
  Constant3/1 -> Bus Creator2/2  "gain"
  Bus Creator2/1 -> Bus Creator1/3  "z"
  Constant2/1 -> Bus Creator2/1  "offset"
  Bus Creator3/1 -> Bus Creator1/2  "y"
  Bus Creator/1 -> Bus Creator1/4  "vx"
  Bus Creator4/1 -> Bus Creator1/1  "x"
  Ramp/1 -> Saturation/1

== system sm_motor_grader_lib/Drawbar/Actuator/Position ==
  q : Inport
  Abs : Abs  ZeroCross=off  SaturateOnIntegerOverflow=off
  PS-Simulink Converter : nesl_utility/PS-Simulink Converter  PhysicalDomain=network_engine_domain  SubClassName=ps_output  LeftPortType=input  RightPortType=output  PseudoPeriodic=off  Frequencies=[]  VectorFormat=inherit  Unit=inherit  AffineConversion=off
  PS-Simulink Converter1 : nesl_utility/PS-Simulink Converter  PhysicalDomain=network_engine_domain  SubClassName=ps_output  LeftPortType=input  RightPortType=output  PseudoPeriodic=off  Frequencies=[]  VectorFormat=inherit  Unit=inherit  AffineConversion=off
  PS-Simulink Converter2 : nesl_utility/PS-Simulink Converter  PhysicalDomain=network_engine_domain  SubClassName=ps_output  LeftPortType=input  RightPortType=output  PseudoPeriodic=off  Frequencies=[]  VectorFormat=inherit  Unit=inherit  AffineConversion=off
  Product : Product
  Revolute Pinion : sm_lib/Joints/Revolute Joint  JointMode=Normal  CompositeWrenchDir=FollowerOnBase  CompositeWrenchFrame=BaseFrame  SenseConstraintForce=off  SenseConstraintTorque=off  SenseTotalForce=off  SenseTotalTorque=off  PositionTargetSpecify=on  PositionTargetPriority=High  PositionTargetValue=-3.5-12  PositionTargetValueUnits=deg  VelocityTargetSpecify=off  VelocityTargetPriority=High  VelocityTargetValue=0  VelocityTargetValueUnits=deg/s  EquilibriumPosition=0  EquilibriumPositionUnits=deg  SpringStiffness=0  SpringStiffnessUnits=N*m/deg  DampingCoefficient=0  DampingCoefficientUnits=N*m/(deg/s)  LowerLimitSpecify=off  LowerLimitBound=-90  LowerLimitBoundUnits=deg  LowerLimitStiffness=1e4  LowerLimitStiffnessUnits=N*m/deg  LowerLimitDamping=10  LowerLimitDampingUnits=N*m/(deg/s)  LowerLimitTransitionRegionWidth=0.1  LowerLimitTransitionRegionWidthUnits=deg  UpperLimitSpecify=off  UpperLimitBound=90  UpperLimitBoundUnits=deg  UpperLimitStiffness=1e4  UpperLimitStiffnessUnits=N*m/deg  UpperLimitDamping=10  UpperLimitDampingUnits=N*m/(deg/s)  UpperLimitTransitionRegionWidth=0.1  UpperLimitTransitionRegionWidthUnits=deg  TorqueActuationMode=ComputedTorque  MotionActuationMode=InputMotion  SensePosition=on  SenseVelocity=on  SenseAcceleration=off  SenseTorqueForce=on  SenseLowerLimitTorqueForce=off  SenseUpperLimitTorqueForce=off
  Simulink-PS Converter : nesl_utility/Simulink-PS Converter  PhysicalDomain=network_engine_domain  SubClassName=ps_input  LeftPortType=input  RightPortType=output  PseudoPeriodic=off  Frequencies=[]  NoiseDistribution=none  NoiseParameters=[]  Unit=deg  AffineConversion=off  FilteringAndDerivatives=filter  SimscapeFilterOrder=2  InputFilterTimeConstant=0.01  UdotUserProvided=0
  R : PMIOPort  Side=Left
  B : PMIOPort  Port=2  Side=Left
  F : PMIOPort  Port=3  Side=Right
  Out Bus Element : Outport  PortName=m  Element=power
  Out Bus Element1 : Outport  PortName=m  Element=torque
  Out Bus Element2 : Outport  PortName=m  Element=w
  Out Bus Element3 : Outport  PortName=m  Element=q
  wires:
  q/1 -> Simulink-PS Converter/1
  PS-Simulink Converter2/1 -> Out Bus Element3/1
  Abs/1 -> Out Bus Element/1
  Product/1 -> Abs/1
  PS-Simulink Converter1/1 -> Out Bus Element2/1, Product/1
  PS-Simulink Converter/1 -> Out Bus Element1/1, Product/2
  connections:
  Simulink-PS Converter/RConn1 -- Revolute Pinion/LConn2
  B/RConn1 -- Revolute Pinion/LConn1
  F/RConn1 -- Revolute Pinion/RConn1
  Revolute Pinion/RConn2 -- PS-Simulink Converter2/LConn1
  Revolute Pinion/RConn3 -- PS-Simulink Converter1/LConn1
  Revolute Pinion/RConn4 -- PS-Simulink Converter/LConn1

== system sm_motor_grader_lib/Drawbar/Actuator/Shaft ==
  q : Inport
  Abs : Abs  ZeroCross=off  SaturateOnIntegerOverflow=off
  Mechanical Rotational Reference : fl_lib/Mechanical/Rotational Elements/Mechanical Rotational Reference
  PS-Simulink Converter : nesl_utility/PS-Simulink Converter  PhysicalDomain=network_engine_domain  SubClassName=ps_output  LeftPortType=input  RightPortType=output  PseudoPeriodic=off  Frequencies=[]  VectorFormat=inherit  Unit=inherit  AffineConversion=off
  PS-Simulink Converter1 : nesl_utility/PS-Simulink Converter  PhysicalDomain=network_engine_domain  SubClassName=ps_output  LeftPortType=input  RightPortType=output  PseudoPeriodic=off  Frequencies=[]  VectorFormat=inherit  Unit=inherit  AffineConversion=off
  PS-Simulink Converter2 : nesl_utility/PS-Simulink Converter  PhysicalDomain=network_engine_domain  SubClassName=ps_output  LeftPortType=input  RightPortType=output  PseudoPeriodic=off  Frequencies=[]  VectorFormat=inherit  Unit=inherit  AffineConversion=off
  Product : Product
  Revolute Pinion : sm_lib/Joints/Revolute Joint  JointMode=Normal  CompositeWrenchDir=FollowerOnBase  CompositeWrenchFrame=BaseFrame  SenseConstraintForce=off  SenseConstraintTorque=off  SenseTotalForce=off  SenseTotalTorque=off  PositionTargetSpecify=on  PositionTargetPriority=High  PositionTargetValue=-3.5-12  PositionTargetValueUnits=deg  VelocityTargetSpecify=off  VelocityTargetPriority=High  VelocityTargetValue=0  VelocityTargetValueUnits=deg/s  EquilibriumPosition=0  EquilibriumPositionUnits=deg  SpringStiffness=0  SpringStiffnessUnits=N*m/deg  DampingCoefficient=0  DampingCoefficientUnits=N*m/(deg/s)  LowerLimitSpecify=off  LowerLimitBound=-90  LowerLimitBoundUnits=deg  LowerLimitStiffness=1e4  LowerLimitStiffnessUnits=N*m/deg  LowerLimitDamping=10  LowerLimitDampingUnits=N*m/(deg/s)  LowerLimitTransitionRegionWidth=0.1  LowerLimitTransitionRegionWidthUnits=deg  UpperLimitSpecify=off  UpperLimitBound=90  UpperLimitBoundUnits=deg  UpperLimitStiffness=1e4  UpperLimitStiffnessUnits=N*m/deg  UpperLimitDamping=10  UpperLimitDampingUnits=N*m/(deg/s)  UpperLimitTransitionRegionWidth=0.1  UpperLimitTransitionRegionWidthUnits=deg  TorqueActuationMode=InputTorque  MotionActuationMode=ComputedMotion  SensePosition=on  SenseVelocity=on  SenseAcceleration=off  SenseTorqueForce=on  SenseLowerLimitTorqueForce=off  SenseUpperLimitTorqueForce=off
  Rotational Multibody Interface : fl_lib/Mechanical/Multibody Interfaces/Rotational Multibody Interface
  Terminator : Terminator
  R : PMIOPort  Side=Left
  B : PMIOPort  Port=2  Side=Left
  F : PMIOPort  Port=3  Side=Right
  Out Bus Element : Outport  PortName=m  Element=power
  Out Bus Element1 : Outport  PortName=m  Element=torque
  Out Bus Element2 : Outport  PortName=m  Element=w
  Out Bus Element3 : Outport  PortName=m  Element=q
  wires:
  PS-Simulink Converter/1 -> Out Bus Element1/1, Product/2
  PS-Simulink Converter1/1 -> Product/1, Out Bus Element2/1
  Product/1 -> Abs/1
  Abs/1 -> Out Bus Element/1
  PS-Simulink Converter2/1 -> Out Bus Element3/1
  q/1 -> Terminator/1
  connections:
  Revolute Pinion/RConn4 -- PS-Simulink Converter/LConn1
  Revolute Pinion/RConn3 -- Rotational Multibody Interface/RConn1 -- PS-Simulink Converter1/LConn1
  Revolute Pinion/RConn2 -- PS-Simulink Converter2/LConn1
  F/RConn1 -- Revolute Pinion/RConn1
  B/RConn1 -- Revolute Pinion/LConn1
  Rotational Multibody Interface/RConn2 -- R/RConn1
  Rotational Multibody Interface/LConn2 -- Mechanical Rotational Reference/LConn1
  Rotational Multibody Interface/LConn1 -- Revolute Pinion/LConn2

== system sm_motor_grader_lib/Frame Front/Knuckle L/Knuckle Lean ==
  LeftLeanKnuckle : sm_lib/Body Elements/File Solid  ExtGeomFileName=LeftFrontLeanKnuckle.step  UnitType=FromFile  ExtGeomFileUnits=m  StepReaderType=HEX  ExportConvexHullGeometry=off  InertiaType=CalculateFromGeometry  BasedOnType=Mass  Density=1000  DensityUnits=kg/m^3  Mass=motGradParams.wheelLeanKnuckle.mass  MassUnits=kg  CenterOfMass=[0 0 0]  CenterOfMassUnits=m  MomentsOfInertia=[1 1 1]  MomentsOfInertiaUnits=kg*m^2  ProductsOfInertia=[0 0 0]  ProductsOfInertiaUnits=kg*m^2  GraphicType=FromGeometry  MarkerShape=Sphere  MarkerSize=10  GraphicVisPropType=SimpleVisualProperties  GraphicDiffuseColor=mtrgrd.clr.knuckle_lean  GraphicOpacity=1  GraphicSpecularColor=[0.5 0.5 0.5 1.0]  GraphicAmbientColor=[0.15 0.15 0.15 1.0]  GraphicEmissiveColor=[0.0 0.0 0.0 1.0]  GraphicShininess=75  DoExposeReferenceFrame=off  SerializedFrames=<Frames><Frame><Id>Frame1</Id><Value><Name>FrontAxle</Name><Origin><Source>GeometricFeature</Source><FeatureName>circular curve 16</FeatureName></Origin><PrimaryAxis><DefinedDirection>+Z</DefinedDirection><Source>GeometricFeature</Source><SourceDirection>+Y</SourceDirection><FeatureName>segment 78</FeatureName></PrimaryAxis><SecondaryAxis><DefinedDirection>+X</DefinedDirection><Source>ReferenceFrame</Source><SourceDirection>+X</SourceDirection><FeatureName></FeatureName></SecondaryAxis></Value></Frame><Frame><Id>Frame2</Id><Value><Name>LeanRod</Name><Origin><Source>GeometricFeature</Source><FeatureName>circular curve 47</FeatureName></Origin><PrimaryAxis><DefinedDirection>+Z</DefinedDirection><Source>GeometricFeature</Source><SourceDirection>+Y</SourceDirection><FeatureName>segment 62</FeatureName></PrimaryAxis><SecondaryAxis><DefinedDirection>+X</DefinedDirection><Source>ReferenceFrame</Source><SourceDirection>+X</SourceDirection><FeatureName></FeatureName></SecondaryAxis></Value></Frame><Frame><Id>Frame3</Id><Value><Name>SteerKnuckle</Name><Origin><Source>GeometricFeature</Source><FeatureName>circular curve 51</FeatureName></Origin><PrimaryAxis><DefinedDirection>-Z</DefinedDirection><Source>GeometricFeature</Source><SourceDirection>+Z</SourceDirection><FeatureName>segment 73</FeatureName></PrimaryAxis><SecondaryAxis><DefinedDirection>+X</DefinedDirection><Source>GeometricFeature</Source><SourceDirection>+X</SourceDirection><FeatureName>segment 13</FeatureName></SecondaryAxis></Value></Frame></Frames>
  Transform Lean Cyl Joint : sm_lib/Frames and Transforms/Rigid Transform  RotationMethod=StandardAxis  FollAlignAxisA=+X  BaseAlignAxisA=+Y  FollAlignAxisB=+Y  BaseAlignAxisB=+Z  RotationStandardAxis=+Y  RotationAngle=90  RotationAngleUnits=deg  RotationArbitraryAxis=[0 0 1]  RotationSequenceAxes=FollowerAxes  RotationSequence=XYX  RotationSequenceAngles=[0 0 0]  RotationSequenceAnglesUnits=deg  RotationMatrix=[1 0 0;0 1 0;0 0 1]  Quaternion=[1 0 0 0]  TranslationMethod=None  TranslationCartesianOffset=[0 0 0]  TranslationCartesianOffsetUnits=m  TranslationStandardAxis=+Z  TranslationStandardOffset=0  TranslationStandardOffsetUnits=m  TranslationROffset=0  TranslationROffsetUnits=m  TranslationThetaOffset=0  TranslationThetaOffsetUnits=deg  TranslationZOffset=0  TranslationZOffsetUnits=m
  Lean Cyl : PMIOPort  Side=Left
  Axle : PMIOPort  Port=2  Side=Left
  Steer : PMIOPort  Port=3  Side=Right
  connections:
  LeftLeanKnuckle/LConn2 -- Steer/RConn1
  Transform Lean Cyl Joint/LConn1 -- LeftLeanKnuckle/RConn1
  LeftLeanKnuckle/LConn1 -- Axle/RConn1
  Lean Cyl/RConn1 -- Transform Lean Cyl Joint/RConn1
